simulink model "AverageCalculator"  (R2021a)
settings: Solver=FixedStepDiscrete  StartTime=0.0  StopTime=10.0  RelTol=1e-3  EnableMultiTasking=on
settings Model: Creator=top one  LastModifiedBy=top one
settings DataIOCC: ReturnWorkspaceOutputs=off
settings OptimizationCC: DefaultParameterBehavior=Inlined  InlineInvariantSignals=on  EnableMemcpy=off  LifeSpan=1  EfficientTunableParamExpr=on
settings DebuggingCC: UnderspecifiedInitializationDetection=Classic  MergeDetectMultiDrivingBlocksExec=none  SFMachineParentedDataDiag=warning  ArithmeticOperatorsInVariantConditions=warning
settings ModelReferenceCC: PropagateSignalLabelsOutOfModel=off
settings SFSimCC: MATLABDynamicMemAlloc=off  CustomCodeUndefinedFunction=UseInterfaceOnly
settings RTWCC: SystemTargetFile=ert.tlc  GenCodeOnly=on  TemplateMakefile=ert_default_tmf  GenerateReport=on  IncludeHyperlinkInReport=on  LaunchReport=on  GenerateTraceInfo=on  GenerateTraceReport=on  GenerateTraceReportSl=on  GenerateTraceReportSf=on  GenerateTraceReportEml=on
settings CodeAppCC: ForceParamTrailComments=on  IgnoreCustomStorageClasses=off  OperatorAnnotations=on  SimulinkDataObjDesc=on  SFDataObjDesc=on  MATLABFcnDesc=on  InsertBlockDesc=on  StateflowObjectComments=on  MATLABSourceComments=on
settings ERTTargetCC: MultiwordLength=2048  GenerateSampleERTMain=on  InlinedParameterPlacement=NonHierarchical  ERTCustomFileTemplate=example_file_process.tlc

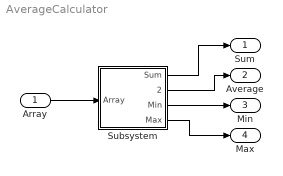
== system AverageCalculator ==
  Array : Inport
  Subsystem : Subsystem
  Sum : Outport
  Average : Outport  Port=2
  Min : Outport  Port=3
  Max : Outport  Port=4
  wires:
  Subsystem/1(Sum) -> Sum/1
  Subsystem/3(Min) -> Min/1
  Subsystem/4(Max) -> Max/1
  Subsystem/2(Average) -> Average/1
  Array/1 -> Subsystem/1(Array)

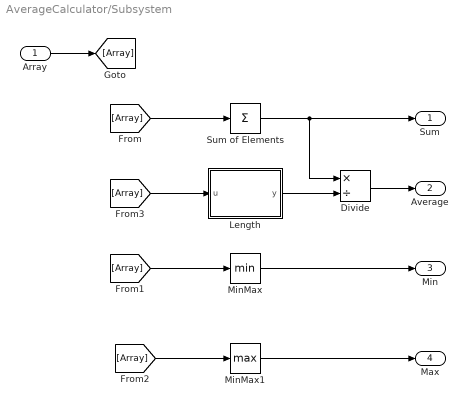
== system AverageCalculator/Subsystem ==
  Array : Inport
  Divide : Product  Inputs=*/
  Length : MATLAB Function  TreatAsAtomicUnit=on
  MinMax : MinMax
  MinMax1 : MinMax  Function=max
  Sum of Elements : Sum  Inputs=+
  Sum : Outport
  Average : Outport  Port=2
  Min : Outport  Port=3
  Max : Outport  Port=4
  wires:
  MinMax1/1 -> Max/1
  [Array] -> Sum of Elements/1
  [Array] -> MinMax1/1
  MinMax/1 -> Min/1
  Sum of Elements/1 -> Divide/1, Sum/1
  Array/1 -> [Array]
  [Array] -> MinMax/1
  [Array] -> Length/1(u)
  Divide/1 -> Average/1
  Length/1(y) -> Divide/2

== matlab function AverageCalculator/Subsystem/Length ==
  data: u input; y output
function y = fcn(u)

y=length(u);
